simulink subsystem "ThreeAxesSignals"  (R2021a)
settings: Solver=VariableStepAuto  StartTime=0.0  StopTime=10.0  RelTol=1e-3
undefined symbols (not defined in the file): euler0, t0x, t0y, t0z, tfx, tfy, tfz
libraries: simulink x6, dspsigops x1
settings Model: Creator=Laura  LastModifiedBy=Laura

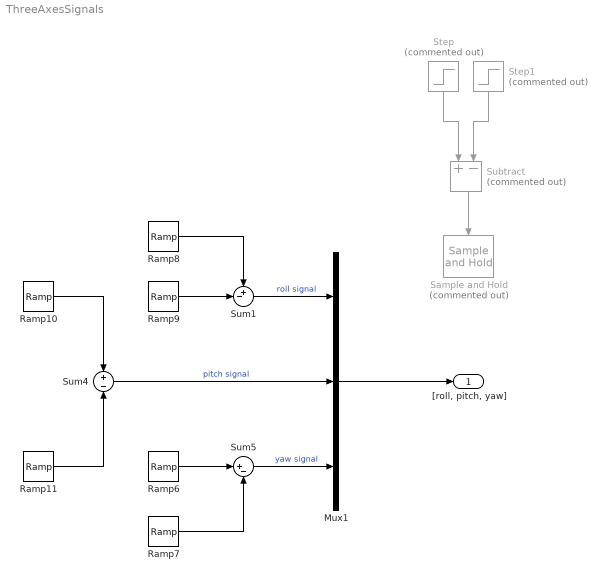
== system ThreeAxesSignals ==
  Mux1 : Mux  Inputs=3
  Ramp10 : simulink/Sources/Ramp  slope=-euler0(2)/(tfy - t0y)  start=t0y  InitialOutput=euler0(2)
  Ramp11 : simulink/Sources/Ramp  slope=-euler0(2)/(tfy - t0y)  start=tfy  InitialOutput=0
  Ramp6 : simulink/Sources/Ramp  slope=-euler0(3)/(tfz - t0z)  start=t0z  InitialOutput=euler0(3)
  Ramp7 : simulink/Sources/Ramp  slope=-euler0(3)/(tfz - t0z)  start=tfz  InitialOutput=0
  Ramp8 : simulink/Sources/Ramp  slope=-euler0(1)/(tfx - t0x)  start=t0x  InitialOutput=euler0(1)
  Ramp9 : simulink/Sources/Ramp  slope=-euler0(1)/(tfx - t0x)  start=tfx  InitialOutput=0
  Sample and Hold : dspsigops/Sample and Hold  Commented=on  trig=Rising edge  initCond=0  latchinput=off
  Step : Step  Commented=on  Time=0.001  SampleTime=0
  Step1 : Step  Commented=on  Time=0.2  SampleTime=0
  Subtract : Sum  Commented=on  Inputs=+-
  Sum1 : Sum  Inputs=+-|
  Sum4 : Sum  Inputs=+-
  Sum5 : Sum  Inputs=|+-
  "[roll, pitch, yaw]" : Outport
  wires:
  Mux1/1 -> "[roll, pitch, yaw]"/1
  Subtract/1 -> Sample and Hold/Trigger
  Step/1 -> Subtract/1
  Step1/1 -> Subtract/2
  Sum5/1 -> Mux1/3  "yaw signal"
  Ramp10/1 -> Sum4/1
  Ramp9/1 -> Sum1/2
  Sum4/1 -> Mux1/2  "pitch signal"
  Ramp8/1 -> Sum1/1
  Ramp11/1 -> Sum4/2
  Ramp7/1 -> Sum5/2
  Ramp6/1 -> Sum5/1
  Sum1/1 -> Mux1/1  "roll signal"
